simulink model "Sim_model"  (Simulink 7.4)
settings: Solver=ode45  StartTime=0.0  StopTime=10  RelTol=1e-6
settings Model: Creator=Lluís  LastModifiedBy=Lluís

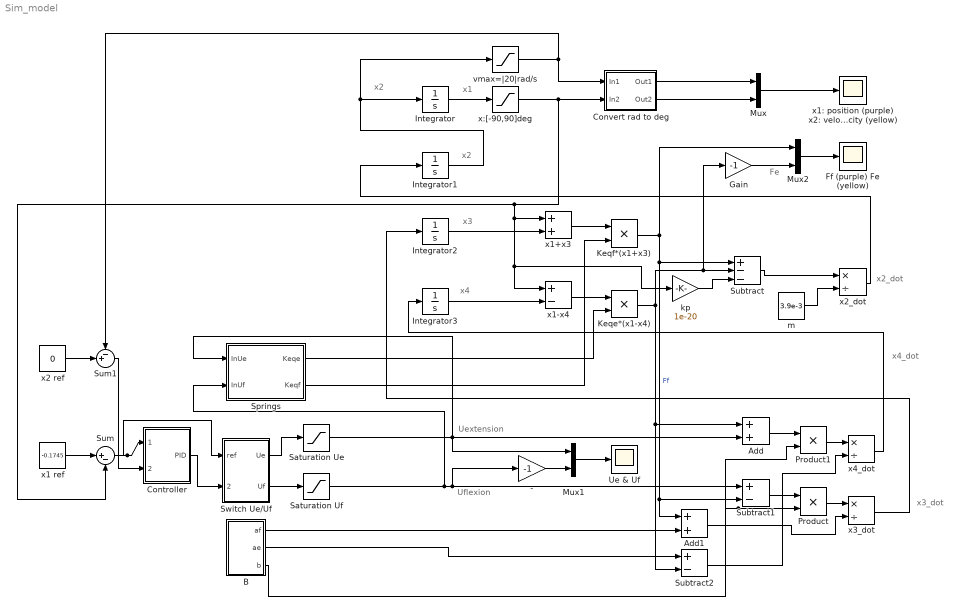
== system Sim_model ==
  note: x2_dot
  note: x4
  note: x3
  note: x2
  note: x1
  note: x2
  note: Uextension
  note: Uflexion
  note: x3_dot
  note: x4_dot
  note: Fe
  - : Gain  Gain=-1  ParameterDataType=fixdt(1, 16)  ParameterScaling=2^0  OutDataType=fixdt(1, 16)  OutScaling=2^0
  Add : Sum  OutDataType=fixdt(1, 16)  OutScaling=2^-10
  Add1 : Sum  OutDataType=fixdt(1, 16)  OutScaling=2^-10
  B : Subsystem
  Controller : Subsystem
  Convert rad to deg : Subsystem
  Ff (purple) Fe (yellow) : Scope
      settings: YMin=-0.1  YMax=2.1  SaveName=ScopeData8
  Gain : Gain  Gain=-1  ParameterDataType=fixdt(1, 16)  ParameterScaling=2^0  OutDataType=fixdt(1, 16)  OutScaling=2^0
  Integrator : Integrator  InitialCondition=0.1745
  Integrator1 : Integrator  InitialCondition=-0.001
  Integrator2 : Integrator
  Integrator3 : Integrator
  Keqe*(x1-x4) : Product  OutDataType=fixdt(1, 16)  OutScaling=2^0  RndMeth=Zero
  Keqf*(x1+x3) : Product  OutDataType=fixdt(1, 16)  OutScaling=2^0  RndMeth=Zero
  Mux : Mux  Inputs=2
  Mux1 : Mux  Inputs=2
  Mux2 : Mux  Inputs=2
  Product : Product  OutDataType=fixdt(1, 16)  OutScaling=2^0  RndMeth=Zero
  Product1 : Product  OutDataType=fixdt(1, 16)  OutScaling=2^0  RndMeth=Zero
  Saturation Ue : Saturate  UpperLimit=12.5  LowerLimit=0  OutDataType=fixdt(1, 16)  OutScaling=2^0
  Saturation Uf : Saturate  UpperLimit=21  LowerLimit=0  OutDataType=fixdt(1, 16)  OutScaling=2^0
  Springs : Subsystem
  Subtract : Sum  Inputs=+--  OutDataType=fixdt(1, 16)  OutScaling=2^-10
  Subtract1 : Sum  Inputs=+-  OutDataType=fixdt(1, 16)  OutScaling=2^-10
  Subtract2 : Sum  Inputs=+-  OutDataType=fixdt(1, 16)  OutScaling=2^-10
  Sum : Sum  Inputs=|+-  OutDataType=fixdt(1, 16)  OutScaling=2^0
  Sum1 : Sum  Inputs=-+|  OutDataType=fixdt(1, 16)  OutScaling=2^0
  Switch Ue/Uf : Subsystem
  Ue & Uf : Scope
  kp : Gain  Gain=1e-20  ParameterDataType=fixdt(1, 16)  ParameterScaling=2^0  OutDataType=fixdt(1, 16)  OutScaling=2^0
  m : Constant  Value=3.9e-3  OutDataType=fixdt(1, 16)  OutScaling=2^0
  vmax=|20|rad/s : Saturate  UpperLimit=1145  LowerLimit=-1145  OutDataType=fixdt(1, 16)  OutScaling=2^0
  x1 ref : Constant  Value=-0.1745  OutDataType=fixdt(1, 16)  OutScaling=2^0
  x1+x3 : Sum  OutDataType=fixdt(1, 16)  OutScaling=2^-10
  x1-x4 : Sum  Inputs=+-  OutDataType=fixdt(1, 16)  OutScaling=2^-10
  x1: position (purple) x2: velocity (yellow) : Scope
      settings: YMin=-0.1  YMax=2.1  SaveName=data  DataFormat=Array
  x2 ref : Constant  Value=0  OutDataType=fixdt(1, 16)  OutScaling=2^0
  x2_dot : Product  Inputs=*/  OutDataType=fixdt(1, 16)  OutScaling=2^-10
  x3_dot : Product  Inputs=*/  OutDataType=fixdt(1, 16)  OutScaling=2^-10
  x4_dot : Product  Inputs=*/  OutDataType=fixdt(1, 16)  OutScaling=2^-10
  x:[-90,90]deg : Saturate  UpperLimit=90/180*pi()  LowerLimit=-90/180*pi()  OutDataType=fixdt(1, 16)  OutScaling=2^0
  wires:
  Mux/1 -> x1: position (purple) x2: velocity (yellow)/1
  Springs/2(Keqf) -> Keqf*(x1+x3)/2
  Springs/1(Keqe) -> Keqe*(x1-x4)/2
  B/2(ae) -> Subtract2/1
  B/1(af) -> Add1/2
  x4_dot/1 -> Integrator3/1
  x3_dot/1 -> Integrator2/1
  x2_dot/1 -> Integrator1/1
  m/1 -> x2_dot/2
  Subtract/1 -> x2_dot/1
  Keqe*(x1-x4)/1 -> Add/1, Subtract2/2, Subtract/2, Gain/1
  Keqf*(x1+x3)/1 -> Subtract/1, Subtract1/2, Add1/1, Mux2/1  "Ff"
  x1-x4/1 -> Keqe*(x1-x4)/1
  x1+x3/1 -> Keqf*(x1+x3)/1
  Integrator2/1 -> x1+x3/2
  Integrator3/1 -> x1-x4/2
  Integrator1/1 -> Integrator/1, vmax=|20|rad/s/1
  Integrator/1 -> x:[-90,90]deg/1
  x1 ref/1 -> Sum/1
  Sum/1 -> Controller/1(ref x1), Switch Ue/Uf/1(ref)
  Mux1/1 -> Ue & Uf/1
  Switch Ue/Uf/1(Ue) -> Saturation Ue/1
  Saturation Ue/1 -> Mux1/1, Springs/1(InUe), Add/2
  Saturation Uf/1 -> Springs/2(InUf), Subtract1/1, -/1
  Switch Ue/Uf/2(Uf) -> Saturation Uf/1
  Subtract1/1 -> Product/1
  B/3(b) -> Product/2, Product1/2
  Product/1 -> x3_dot/1
  Add/1 -> Product1/1
  Product1/1 -> x4_dot/1
  Add1/1 -> x3_dot/2
  Subtract2/1 -> x4_dot/2
  Convert rad to deg/1(Out1) -> Mux/1
  Convert rad to deg/2(Out2) -> Mux/2
  x:[-90,90]deg/1 -> x1+x3/1, x1-x4/1, kp/1, Sum/2, Convert rad to deg/2(In2)
  x2 ref/1 -> Sum1/2
  Sum1/1 -> Controller/2(ref x2)
  Controller/1(PID) -> Switch Ue/Uf/2(control)
  -/1 -> Mux1/2
  kp/1 -> Subtract/3
  vmax=|20|rad/s/1 -> Convert rad to deg/1(In1), Sum1/1
  Gain/1 -> Mux2/2
  Mux2/1 -> Ff (purple) Fe (yellow)/1

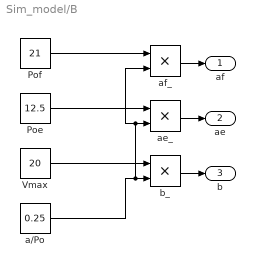
== system Sim_model/B ==
  Poe : Constant  Value=12.5  OutDataType=fixdt(1, 16)  OutScaling=2^0
  Pof : Constant  Value=21  OutDataType=fixdt(1, 16)  OutScaling=2^0
  Vmax : Constant  Value=20  OutDataType=fixdt(1, 16)  OutScaling=2^0
  a/Po : Constant  Value=0.25  OutDataType=fixdt(1, 16)  OutScaling=2^0
  ae_ : Product  OutDataType=fixdt(1, 16)  OutScaling=2^0  RndMeth=Zero
  af_ : Product  OutDataType=fixdt(1, 16)  OutScaling=2^0  RndMeth=Zero
  b_ : Product  OutDataType=fixdt(1, 16)  OutScaling=2^0  RndMeth=Zero
  af : Outport
  ae : Outport  Port=2
  b : Outport  Port=3
  wires:
  Pof/1 -> af_/1
  a/Po/1 -> af_/2, ae_/2, b_/2
  Poe/1 -> ae_/1
  Vmax/1 -> b_/1
  af_/1 -> af/1
  ae_/1 -> ae/1
  b_/1 -> b/1

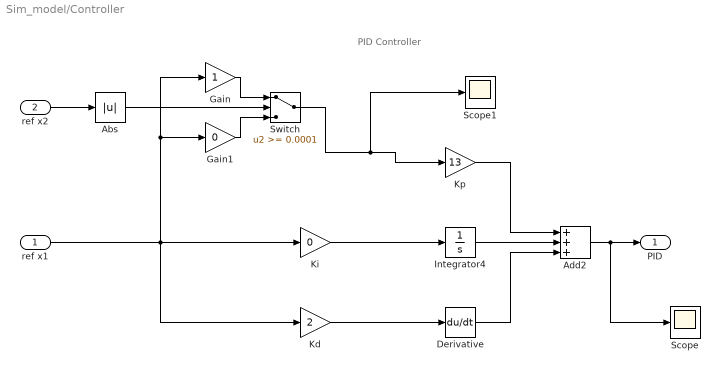
== system Sim_model/Controller ==
  note: PID Controller
  ref x1 : Inport  OutDataType=fixdt(1, 16)  OutScaling=2^0
  ref x2 : Inport  Port=2  OutDataType=fixdt(1, 16)  OutScaling=2^0
  Abs : Abs  OutDataType=fixdt(1, 16)  OutScaling=2^0
  Add2 : Sum  Inputs=+++  OutDataType=fixdt(1, 16)  OutScaling=2^-10
  Derivative : Derivative
  Gain : Gain  ParameterDataType=fixdt(1, 16)  ParameterScaling=2^0  OutDataType=fixdt(1, 16)  OutScaling=2^0
  Gain1 : Gain  Gain=0  ParameterDataType=fixdt(1, 16)  ParameterScaling=2^0  OutDataType=fixdt(1, 16)  OutScaling=2^0
  Integrator4 : Integrator
  Kd : Gain  Gain=2  ParameterDataType=fixdt(1, 16)  ParameterScaling=2^0  OutDataType=fixdt(1, 16)  OutScaling=2^0
  Ki : Gain  Gain=0  ParameterDataType=fixdt(1, 16)  ParameterScaling=2^0  OutDataType=fixdt(1, 16)  OutScaling=2^0
  Kp : Gain  Gain=13  ParameterDataType=fixdt(1, 16)  ParameterScaling=2^0  OutDataType=fixdt(1, 16)  OutScaling=2^0
  Scope : Scope
      settings: SaveName=ScopeData2
  Scope1 : Scope
      settings: SaveName=ScopeData7
  Switch : Switch  Threshold=0.0001  OutDataType=fixdt(1, 16)  OutScaling=2^0
  PID : Outport
  wires:
  ref x1/1 -> Ki/1, Kd/1, Gain/1, Gain1/1
  Add2/1 -> PID/1, Scope/1
  Kp/1 -> Add2/1
  Derivative/1 -> Add2/3
  Kd/1 -> Derivative/1
  Ki/1 -> Integrator4/1
  Integrator4/1 -> Add2/2
  ref x2/1 -> Abs/1
  Gain/1 -> Switch/1
  Gain1/1 -> Switch/3
  Abs/1 -> Switch/2
  Switch/1 -> Kp/1, Scope1/1

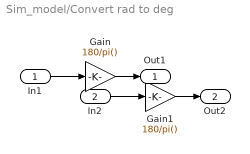
== system Sim_model/Convert rad to deg ==
  In1 : Inport
  In2 : Inport  Port=2
  Gain : Gain  Gain=180/pi()  ParameterDataType=fixdt(1, 16)  ParameterScaling=2^0  OutDataType=fixdt(1, 16)  OutScaling=2^0
  Gain1 : Gain  Gain=180/pi()  ParameterDataType=fixdt(1, 16)  ParameterScaling=2^0  OutDataType=fixdt(1, 16)  OutScaling=2^0
  Out1 : Outport
  Out2 : Outport  Port=2
  wires:
  In1/1 -> Gain/1
  In2/1 -> Gain1/1
  Gain/1 -> Out1/1
  Gain1/1 -> Out2/1

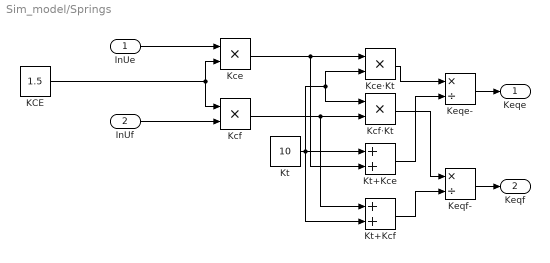
== system Sim_model/Springs ==
  InUe : Inport  OutDataType=fixdt(1, 16)  OutScaling=2^0
  InUf : Inport  Port=2  OutDataType=fixdt(1, 16)  OutScaling=2^0
  KCE : Constant  Value=1.5  OutDataType=fixdt(1, 16)  OutScaling=2^0
  Kce : Product  OutDataType=fixdt(1, 16)  OutScaling=2^0  RndMeth=Zero
  Kce·Kt : Product  OutDataType=fixdt(1, 16)  OutScaling=2^0  RndMeth=Zero
  Kcf : Product  OutDataType=fixdt(1, 16)  OutScaling=2^0  RndMeth=Zero
  Kcf·Kt : Product  OutDataType=fixdt(1, 16)  OutScaling=2^0  RndMeth=Zero
  Keqe- : Product  Inputs=*/  OutDataType=fixdt(1, 16)  OutScaling=2^-10
  Keqf- : Product  Inputs=*/  OutDataType=fixdt(1, 16)  OutScaling=2^-10
  Kt : Constant  Value=10  OutDataType=fixdt(1, 16)  OutScaling=2^0
  Kt+Kce : Sum  OutDataType=fixdt(1, 16)  OutScaling=2^-10
  Kt+Kcf : Sum  OutDataType=fixdt(1, 16)  OutScaling=2^-10
  Keqe : Outport
  Keqf : Outport  Port=2
  wires:
  KCE/1 -> Kce/2, Kcf/1
  Kcf/1 -> Kcf·Kt/2, Kt+Kcf/1
  Kce/1 -> Kce·Kt/1, Kt+Kce/2
  Kt/1 -> Kce·Kt/2, Kcf·Kt/1, Kt+Kce/1, Kt+Kcf/2
  Kce·Kt/1 -> Keqe-/1
  Kt+Kce/1 -> Keqe-/2
  Kcf·Kt/1 -> Keqf-/1
  Kt+Kcf/1 -> Keqf-/2
  Keqe-/1 -> Keqe/1
  Keqf-/1 -> Keqf/1
  InUe/1 -> Kce/1
  InUf/1 -> Kcf/2

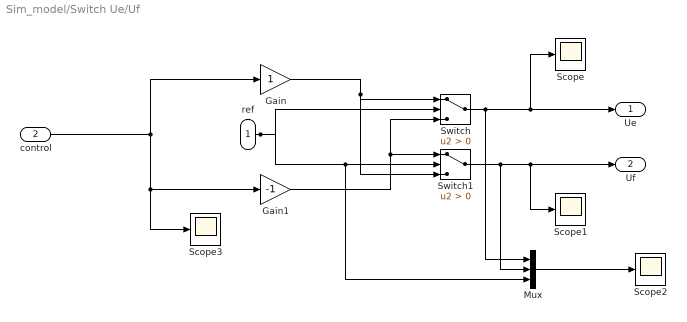
== system Sim_model/Switch Ue/Uf ==
  ref : Inport
  control : Inport  Port=2  OutDataType=fixdt(1, 16)  OutScaling=2^0
  Gain : Gain  ParameterDataType=fixdt(1, 16)  ParameterScaling=2^0  OutDataType=fixdt(1, 16)  OutScaling=2^0
  Gain1 : Gain  Gain=-1  ParameterDataType=fixdt(1, 16)  ParameterScaling=2^0  OutDataType=fixdt(1, 16)  OutScaling=2^0
  Mux : Mux  Inputs=3
  Scope{,1..3} (4 alike) : Scope
      Scope settings: SaveName=ScopeData3
      Scope1 settings: SaveName=ScopeData4
      Scope2 settings: SaveName=ScopeData6
      Scope3 settings: SaveName=ScopeData5
  Switch : Switch  Criteria=u2 > Threshold  OutDataType=fixdt(1, 16)  OutScaling=2^0
  Switch1 : Switch  Criteria=u2 > Threshold  OutDataType=fixdt(1, 16)  OutScaling=2^0
  Ue : Outport
  Uf : Outport  Port=2
  wires:
  ref/1 -> Switch/2, Switch1/2, Mux/3
  Switch/1 -> Ue/1, Scope/1, Mux/1
  Switch1/1 -> Uf/1, Scope1/1, Mux/2
  Gain/1 -> Switch/1, Switch1/3
  Gain1/1 -> Switch/3, Switch1/1
  Mux/1 -> Scope2/1
  control/1 -> Gain/1, Gain1/1, Scope3/1
